simulink model "AutoSizeOnConnectTest"  (Simulink 8.0)
settings: Solver=ode45  StartTime=0.0  StopTime=10.0  RelTol=1e-3
settings Model: Creator=manthony  LastModifiedBy=manthony
settings DataIOCC: SignalLoggingSaveFormat=ModelDataLogs
settings DebuggingCC: FcnCallInpInsideContextMsg=UseLocalSettings
settings GRTTargetCC: CombineOutputUpdateFcns=off  GRTInterface=on

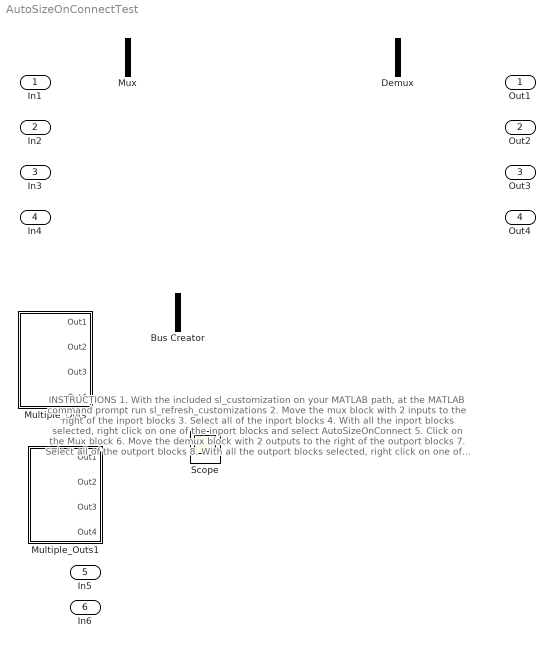
== system AutoSizeOnConnectTest ==
  note: INSTRUCTIONS
      | 1. With the included sl_customization on your MATLAB path, at the
      |     MATLAB command prompt run sl_refresh_customizations
      | 2. Move the mux block with 2 inputs to the right of the inport blocks
      | 3. Select all of the inport blocks
      | 4. With all the inport blocks selected, right click on one of the inport
      |     blocks and select AutoSizeOnConnect
      | 5. Click on the Mux block
      |
      | 6. Move the demux block with 2 outputs to the right of the outport blocks
      | 7. Select all of the outport blocks
      | 8. With all the outport blocks selected, right click on one of the outport
      |     blocks and select AutoSizeOnConnect
      | 9. Click on the Demux block
      |
      | 10. Select the subsystem Multiple_Outs.
      | 11. Right-click on the subsystem Multple_Outs and select AutoSizeOnConnect
      | 12. Click on the Bus Creator block
      |
      | 13. Select the subsystem Multiple_Outs1 and the inport blocks In5 and In6.
      | 14. Right-click and select AutoSizeOnConnect.
      | 15. Click the Scope Block.
      |
      | NOTE: This is also using the AutoSize capability. Without AutoSize, this
      | function will still automatically create the right number of ports for the
      | mux/demux, but will not resize the block to make the lines straight.
  In1 : Inport
  In2 : Inport  Port=2
  In3 : Inport  Port=3
  In4 : Inport  Port=4
  In5 : Inport  Port=5
  In6 : Inport  Port=6
  Bus Creator : BusCreator  Inputs=2
      settings: CopyFcn=AutoSize;  MoveFcn=AutoSize;
  Demux : Demux  Outputs=2
      settings: CopyFcn=AutoSize;  MoveFcn=AutoSize;
  Multiple_Outs : Subsystem  TreatAsAtomicUnit=on
  Multiple_Outs1 : Subsystem  TreatAsAtomicUnit=on
  Mux : Mux  Inputs=2
      settings: CopyFcn=AutoSize;  MoveFcn=AutoSize;
  Scope : Scope
  Out1 : Outport
  Out2 : Outport  Port=2
  Out3 : Outport  Port=3
  Out4 : Outport  Port=4

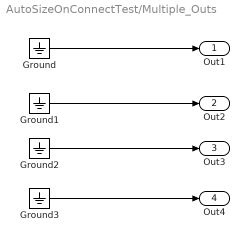
== system AutoSizeOnConnectTest/Multiple_Outs ==
  Ground{,1..3} (4 alike) : Ground
  Out1 : Outport
  Out2 : Outport  Port=2
  Out3 : Outport  Port=3
  Out4 : Outport  Port=4
  wires:
  Ground/1 -> Out1/1
  Ground1/1 -> Out2/1
  Ground2/1 -> Out3/1
  Ground3/1 -> Out4/1

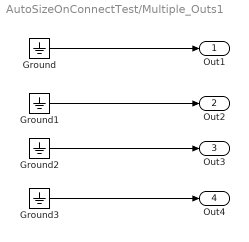
== system AutoSizeOnConnectTest/Multiple_Outs1 ==
  Ground{,1..3} (4 alike) : Ground
  Out1 : Outport
  Out2 : Outport  Port=2
  Out3 : Outport  Port=3
  Out4 : Outport  Port=4
  wires:
  Ground3/1 -> Out4/1
  Ground2/1 -> Out3/1
  Ground1/1 -> Out2/1
  Ground/1 -> Out1/1
